simulink model "BFN_01_Gyro_filter"  (R2019b)
settings: Solver=ode45  StartTime=0.0  StopTime=20  RelTol=1e-6  EnableMultiTasking=on
values from neighbouring files (symbols this model uses):
  Gyro_freq = 1e3    (= 1000)    [BFN_00_main.m]
  Gyro_noise_b = 1/3600*pi/180*sqrt(Gyro_freq)    [BFN_00_main.m]
  Gyro_noise_n = 0.01/60*pi/180*sqrt(Gyro_freq)    [BFN_00_main.m]
  Jsc = [0.0333 0.0838 0.1037]    [BFN_00_main.m]
libraries: dspsrcs4 x2
settings Model: Creator=jsb12221  LastModifiedBy=Nicola
settings DataIOCC: LimitDataPoints=on  SaveFormat=Array  SignalLoggingSaveFormat=ModelDataLogs  ReturnWorkspaceOutputs=off
settings OptimizationCC: ExpressionDepthLimit=2147483647  LifeSpan=inf
settings DebuggingCC: UnderspecifiedInitializationDetection=Classic  MergeDetectMultiDrivingBlocksExec=none  FcnCallInpInsideContextMsg=warning  UnknownTsInhSupMsg=none  StateNameClashWarn=warning  SFUnexpectedBacktrackingDiag=warning  SFNoUnconditionalDefaultTransitionDiag=warning  SFExecutionAtInitializationDiag=none  ArithmeticOperatorsInVariantConditions=warning
settings HardwareCC: ProdBitPerPointer=32  ProdBitPerSizeT=32  ProdBitPerPtrDiffT=32  ProdLargestAtomicFloat=None  ProdIntDivRoundTo=Undefined  ProdEndianess=Unspecified  ProdWordSize=32  ProdHWDeviceType=32-bit Generic
settings ModelReferenceCC: PropagateSignalLabelsOutOfModel=off
settings SFSimCC: SimUseLocalCustomCode=off  CustomCodeUndefinedFunction=UseInterfaceOnly
settings RTWCC: RTWUseLocalCustomCode=off
settings CodeAppCC: StateflowObjectComments=on
settings GRTTargetCC: TargetLangStandard=C89/C90 (ANSI)  GeneratePreprocessorConditionals=Disable all
settings ConfigComp: CovMetricSettings=dw  CovHtmlReporting=on  CovSaveCumulativeToWorkspaceVar=on  CovSaveSingleToWorkspaceVar=on  CovExternalEMLEnable=off

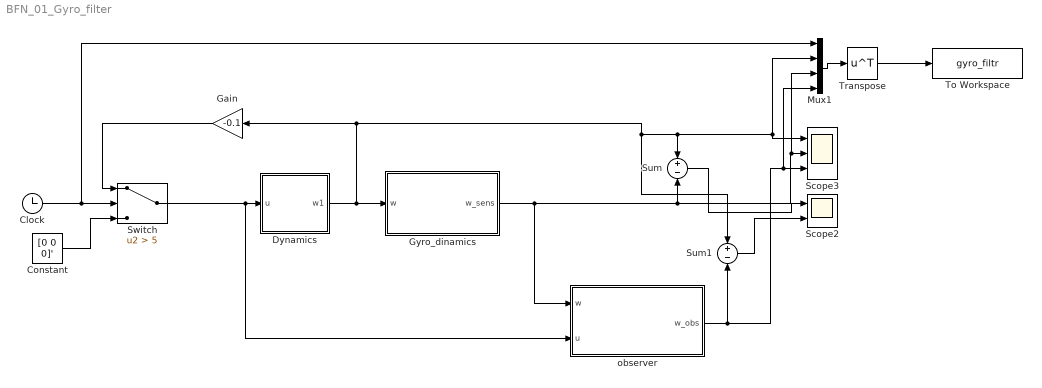
== system BFN_01_Gyro_filter ==
  Clock : Clock
  Constant : Constant  Value=[0 0 0]'
  Dynamics : Subsystem
  Gain : Gain  Gain=-0.1
  Gyro_dinamics : Subsystem
  Mux1 : Mux
  Scope2 : Scope  NumInputPorts=2
  Scope3 : Scope  NumInputPorts=3
  Sum : Sum  Inputs=+-
  Sum1 : Sum  Inputs=+-
  Switch : Switch  Criteria=u2 > Threshold  Threshold=5
  To Workspace : ToWorkspace  VariableName=gyro_filtr  SampleTime=-1
      settings: Save2DSignal=2-D array (concatenate along first dimension)
  Transpose : Math  Operator=transpose  SignedPower=off  SaturateOnIntegerOverflow=on
  observer : Subsystem
  wires:
  Dynamics/1(w1) -> Gyro_dinamics/1(w), Sum1/1, Mux1/2, Scope3/1, Sum/1, Gain/1
  Switch/1 -> observer/2(u), Dynamics/1(u)
  observer/1(w_obs) -> Mux1/4, Scope3/3, Sum1/2
  Sum/1 -> Scope2/1
  Sum1/1 -> Scope2/2
  Gyro_dinamics/1(w_sens) -> observer/1(w), Sum/2, Mux1/3, Scope3/2
  Clock/1 -> Mux1/1, Switch/2
  Constant/1 -> Switch/3
  Gain/1 -> Switch/1
  Mux1/1 -> Transpose/1
  Transpose/1 -> To Workspace/1

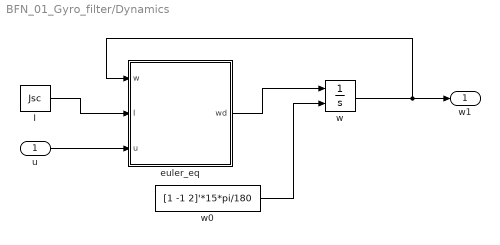
== system BFN_01_Gyro_filter/Dynamics ==
  u : Inport
  I : Constant  Value=Jsc
  euler_eq : MATLAB Function  TreatAsAtomicUnit=on
  w : Integrator  InitialConditionSource=external
  w0 : Constant  Value=[1 -1 2]'*15*pi/180
  w1 : Outport
  wires:
  euler_eq/1(wd) -> w/1
  w0/1 -> w/2
  w/1 -> euler_eq/1(w), w1/1
  I/1 -> euler_eq/2(I)
  u/1 -> euler_eq/3(u)

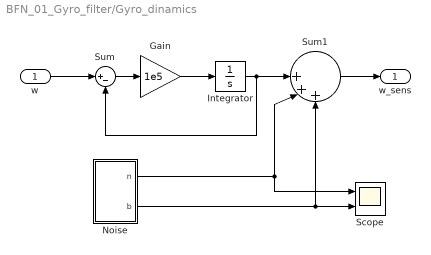
== system BFN_01_Gyro_filter/Gyro_dinamics ==
  w : Inport
  Gain : Gain  Gain=1e5
  Integrator : Integrator  InitialCondition=[0 0 0]'
  Noise : Subsystem
  Scope : Scope  NumInputPorts=2
  Sum : Sum  Inputs=|+-
  Sum1 : Sum  Inputs=||+++
  w_sens : Outport
  wires:
  w/1 -> Sum/1
  Sum/1 -> Gain/1
  Integrator/1 -> Sum/2, Sum1/1
  Gain/1 -> Integrator/1
  Sum1/1 -> w_sens/1
  Noise/1(n) -> Scope/1, Sum1/2
  Noise/2(b) -> Scope/2, Sum1/3

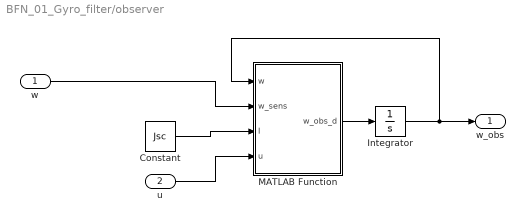
== system BFN_01_Gyro_filter/observer ==
  w : Inport
  u : Inport  Port=2
  Constant : Constant  Value=Jsc
  Integrator : Integrator  InitialCondition=[0 0 0]'
  MATLAB Function : MATLAB Function  TreatAsAtomicUnit=on
  w_obs : Outport
  wires:
  Integrator/1 -> MATLAB Function/1(w), w_obs/1
  MATLAB Function/1(w_obs_d) -> Integrator/1
  u/1 -> MATLAB Function/4(u)
  Constant/1 -> MATLAB Function/3(I)
  w/1 -> MATLAB Function/2(w_sens)

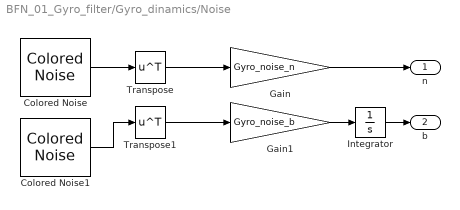
== system BFN_01_Gyro_filter/Gyro_dinamics/Noise ==
  Colored Noise : dspsrcs4/Colored Noise  Color=white  InverseFrequencyPower=1  BoundedOutput=off  NumChannels=3  OutputDataType=double  SamplesPerFrame=1  SampleTime=1/Gyro_freq  RandomStream=mt19937ar with seed  Seed=67  SimulateUsing=Interpreted execution
      settings: SourceProductName=DSP System Toolbox  SourceProductBaseCode=DS
  Colored Noise1 : dspsrcs4/Colored Noise  Color=white  InverseFrequencyPower=1  BoundedOutput=off  NumChannels=3  OutputDataType=double  SamplesPerFrame=1  SampleTime=1/Gyro_freq  RandomStream=mt19937ar with seed  Seed=34  SimulateUsing=Interpreted execution
      settings: SourceProductName=DSP System Toolbox  SourceProductBaseCode=DS
  Gain : Gain  Gain=Gyro_noise_n
  Gain1 : Gain  Gain=Gyro_noise_b
  Integrator : Integrator  InitialCondition=[3 -3 0]'*Gyro_noise_b*1e-2*0
  Transpose : Math  Operator=transpose  SignedPower=off  SaturateOnIntegerOverflow=on
  Transpose1 : Math  Operator=transpose  SignedPower=off  SaturateOnIntegerOverflow=on
  n : Outport
  b : Outport  Port=2
  wires:
  Transpose/1 -> Gain/1
  Integrator/1 -> b/1
  Colored Noise/1 -> Transpose/1
  Gain1/1 -> Integrator/1
  Gain/1 -> n/1
  Transpose1/1 -> Gain1/1
  Colored Noise1/1 -> Transpose1/1

== matlab function BFN_01_Gyro_filter/observer/MATLAB Function ==
  data: w input; w_sens input; I input; u input; w_obs_d output
function w_obs_d = fcn(w,w_sens,I,u)
al = -0.5;
J=diag(I);
w_obs_d = J\(cross(J*w,w)+u+al*(w-w_sens));

== matlab function BFN_01_Gyro_filter/Dynamics/euler_eq ==
  data: w input; wd output; I input; u input
function wd = euler_eq(w,I,u)
J=diag(I);
wd = J\(cross(J*w,w)+u);
